simulink model "FullCardioLablModel"  (R2023b)
settings: Solver=FixedStepDiscrete  StartTime=0.0  StopTime=param_sim_time  FixedStep=1/fs  MaxStep=1/fs  RelTol=1e-3
undefined symbols (not defined in the file): analyses, fdesignblkfcn, fs, gcbh, param_tot_samples
libraries: dspstat3 x13, SCGAnalysis_SignalGenerationLib x2
(part 13 of 20)

== matlab function FullCardioLablModel/SCG Analysis/Enabled SCG Analysis Subsystem/All Signals Signal Metric Characterization/SCG 3DMinS2p2pProjection Signal Metric Characterization/Spectral Distribution Calculator/Spectral Distribution Calculator ==
  data: fs input size=[1]; r_pos input; scg_signal input; entire_cycle_nsd output size=[3 1]; entire_cycle_flag input size=[1]; s1_flag input size=[1]; s2_flag input size=[1]; f_band_lo input size=[1 2]; f_band_mid input size=[1 2]; f_band_hi input size=[1 2]; s1_nsd output size=[3 1]; s2_nsd output size=[3 1]
function [entire_cycle_nsd, s1_nsd, s2_nsd] = slk_normalized_spectral_distribution_calculator(fs, r_pos,scg_signal, entire_cycle_flag, s1_flag, s2_flag, f_band_lo, f_band_mid, f_band_hi)
% Simulink function to calculate the normalized spectral distribution of the power spectral densities of the entire cyle, the s1 complex, and the s2 complex, of an input SCG signal.

% INPUTS:
% fs = sampling frequency of scg_signal.
% r_pos = index positions of the R peaks of the ecg.
% scg_signal = signal to calculate its average cycle.
% entire_cycle_flag = flag to indicate the calculation of the entire cycle spectral distribution.
% s1_flag = flag to indicate the calculation of the S1 complex spectral distribution.
% s2_flag = flag to indicate the calculation of the S2 complex spectral distribution.

% OUTPUT:
% entire_cycle_nsd = normalized spectral distribution of the entire cycle (given as 3 elements corresponding to the spectral distribution in each of the 3 bins).
% s1_nsd = normalized spectral distribution of the s1 complex (given as 3 elements corresponding to the spectral distribution in each of the 3 bins).
% s2_nsd = normalized spectral distribution of the s2 complex (given as 3 elements corresponding to the spectral distribution in each of the 3 bins).

% This function consists of three parts:
% Part 1 - Calculation of the entire cycle normalized spectral distribution.
% Part 2 - Calculation of the S1 complex normalized spectral distribution.
% Part 3 - Calculation of the S2 complex normalized spectral distribution.

coder.extrinsic('legend');
coder.extrinsic('vline');

num_cycles = length(r_pos);

pad_size = 10*fs; % The length of the zero-padded vector used to obtain sufficient frequency resolution for the FFT.

PSDs = figure;
xlabel('Frequency (Hz)')
ylabel('Power Spectral Density (mg^2)')
xlim([0 f_band_hi(2)])
title('Power Spectral Densities')
hold on

freq_axis = fs*(0:pad_size/2)/pad_size; % Frequency axis for the FFT.

%% Part 1 - Calculation of the entire cycle normalized spectral distribution.


% if entire_cycle_flag
%     
%     current_cycle_padded = zeros(pad_size,1); % Pre-initializing for speed.
%     fft_entire_cycle_mag_2_sided = zeros(pad_size,1);
%     fft_entire_cycle_mag_1_sided = zeros(pad_size/2+1,num_cycles - 1);
%     
%     for i = 1:num_cycles - 1 % The last cycle isnt considered because it's not complete.
%         
%         current_cycle = scg_signal(r_pos(i):r_pos(i+1));
%         current_cycle_length = length(current_cycle); % In samples.
%         
%         % Ensuring the current cycle has an even number of samples - necessary for FFT calculation.
%         if mod(current_cycle_length,2) > 0
%             current_cycle_length = current_cycle_length - 1;
%             current_cycle(end) = [];
%         end
%                
%         current_cycle_padded = [current_cycle; zeros(pad_size - current_cycle_length,1)];
%         fft_entire_cycle = fft(current_cycle_padded); % (Complex) FFT values.
%         fft_entire_cycle_mag_2_sided = abs(fft_entire_cycle); % Two-sided Magnitude.
%         fft_entire_cycle_mag_1_sided(:,i) = fft_entire_cycle_mag_2_sided(1:length(current_cycle_padded)/2+1); % One-sided Magnitude.
%         fft_entire_cycle_mag_1_sided(2:end-1,i) = 2*fft_entire_cycle_mag_1_sided(2:end-1,i); % Multiplying by 2 to get total power (negative + positive frequencies).
%     end
%     
%     average_entire_cycle_fft = mean(fft_entire_cycle_mag_1_sided'); % The mean magnitude FFT spectrum.
%     
%     average_entire_cycle_psd = average_entire_cycle_fft.^2; % The power spectral density - the square of the magnitude spectrum.
%     
%     % Plotting.
%     figure(PSDs); hold on;
%     plot(freq_axis,average_entire_cycle_psd)
%     
%     % Integrating along the bands to get the bandpower.
%     entire_cycle_lo_power = trapz(ceil(f_band_lo(1)/freq_axis(2)):ceil(f_band_lo(2)/freq_axis(2)),average_entire_cycle_psd(ceil(f_band_lo(1)/freq_axis(2)):ceil(f_band_lo(2)/freq_axis(2))));
%     entire_cycle_mid_power = trapz(ceil(f_band_mid(1)/freq_axis(2)):ceil(f_band_mid(2)/freq_axis(2)),average_entire_cycle_psd(ceil(f_band_mid(1)/freq_axis(2)):ceil(f_band_mid(2)/freq_axis(2))));
%     entire_cycle_hi_power = trapz(ceil(f_band_hi(1)/freq_axis(2)):ceil(f_band_hi(2)/freq_axis(2)),average_entire_cycle_psd(ceil(f_band_hi(1)/freq_axis(2)):ceil(f_band_hi(2)/freq_axis(2))));
%     entire_cycle_total_power = trapz(ceil(f_band_lo(1)/freq_axis(2)):ceil(f_band_hi(2)/freq_axis(2)),average_entire_cycle_psd(ceil(f_band_lo(1)/freq_axis(2)):ceil(f_band_hi(2)/freq_axis(2))));
%     
%     % Dividing over total power to get the normalized spectral distribution (NSD).
%     normalized_entire_cycle_lo_power = entire_cycle_lo_power/entire_cycle_total_power;
%     normalized_entire_cycle_mid_power = entire_cycle_mid_power/entire_cycle_total_power;
%     normalized_entire_cycle_hi_power = entire_cycle_hi_power/entire_cycle_total_power;
%     
%     % Preparing outputs.
%     entire_cycle_nsd = [normalized_entire_cycle_lo_power;normalized_entire_cycle_mid_power;normalized_entire_cycle_hi_power];
%     
% else 
%     entire_cycle_nsd = [0; 0; 0];
% end


if entire_cycle_flag

    Interp_FFT_Cycle_Mag_1_Sided = zeros(num_cycles - 1, 10000); % Pre-initializing for speed.
    new_freq_axis_entire_cycle = linspace(0,fs/2,10000); % Interpolation frequency axis.

    for i = 1:num_cycles - 1 % The last cycle isnt considered because it's not complete.

        current_cycle = scg_signal(r_pos(i):r_pos(i+1));
        current_cycle_length = length(current_cycle); % In samples.

        % Ensuring the current cycle has an even number of samples - necessary for FFT calculation.
        if mod(current_cycle_length,2) > 0
            current_cycle_length = current_cycle_length - 1;
            current_cycle(end) = [];
        end

        FFT_Cycle = zeros(current_cycle_length,1); % Pre-initializing for speed.
        FFT_Cycle_Mag_2_Sided = zeros(current_cycle_length,1);
        FFT_Cycle_Mag_1_Sided = zeros(current_cycle_length/2+1,1);

        freq_axis_entire_cycle = fs*(0:current_cycle_length/2)/current_cycle_length; % Frequency axis for the FFT.

        % FFT of each individual cycle.
        FFT_Cycle = fft(current_cycle); % (Complex) FFT values.
        FFT_Cycle_Mag_2_Sided = abs(FFT_Cycle); % Two-sided Magnitude.
        FFT_Cycle_Mag_1_Sided = FFT_Cycle_Mag_2_Sided(1:current_cycle_length/2+1); % One-sided Magnitude.
        FFT_Cycle_Mag_1_Sided(2:end-1) = 2*FFT_Cycle_Mag_1_Sided(2:end-1); % Multiplying by 2 to get total power (negative + positive frequencies).

        % Interpolating to a new frequency axis. This is necessary because different cycles have different lenghts (and thus different FFT
        % lengths). To average the FFT across cycles, these must be interpolated to a particular fixed length.
        Interp_FFT_Cycle_Mag_1_Sided(i,:) = interp1(freq_axis_entire_cycle, FFT_Cycle_Mag_1_Sided, new_freq_axis_entire_cycle);

    end

    average_entire_cycle_FFT = mean(Interp_FFT_Cycle_Mag_1_Sided); % The mean magnitude FFT spectrum.

    average_entire_cycle_PSD = average_entire_cycle_FFT.^2; % The power spectral density - the square of the magnitude spectrum.

    % Plotting
    figure(PSDs);
    plot(new_freq_axis_entire_cycle,average_entire_cycle_PSD)

    % Integrating along the bands to get the bandpower.
    entire_cycle_lo_power = trapz(ceil(f_band_lo(1)/new_freq_axis_entire_cycle(2)):ceil(f_band_lo(2)/new_freq_axis_entire_cycle(2)),average_entire_cycle_PSD(ceil(f_band_lo(1)/new_freq_axis_entire_cycle(2)):ceil(f_band_lo(2)/new_freq_axis_entire_cycle(2))));
    entire_cycle_mid_power = trapz(ceil(f_band_mid(1)/new_freq_axis_entire_cycle(2)):ceil(f_band_mid(2)/new_freq_axis_entire_cycle(2)),average_entire_cycle_PSD(ceil(f_band_mid(1)/new_freq_axis_entire_cycle(2)):ceil(f_band_mid(2)/new_freq_axis_entire_cycle(2))));
    entire_cycle_hi_power = trapz(ceil(f_band_hi(1)/new_freq_axis_entire_cycle(2)):ceil(f_band_hi(2)/new_freq_axis_entire_cycle(2)),average_entire_cycle_PSD(ceil(f_band_hi(1)/new_freq_axis_entire_cycle(2)):ceil(f_band_hi(2)/new_freq_axis_entire_cycle(2))));
    entire_cycle_total_power = trapz(ceil(f_band_lo(1)/new_freq_axis_entire_cycle(2)):ceil(f_band_hi(2)/new_freq_axis_entire_cycle(2)),average_entire_cycle_PSD(ceil(f_band_lo(1)/new_freq_axis_entire_cycle(2)):ceil(f_band_hi(2)/new_freq_axis_entire_cycle(2))));

    % Dividing over total power to get the normalized spectral distribution (NSD).
    normalized_entire_cyce_lo_power = entire_cycle_lo_power/entire_cycle_total_power;
    normalized_entire_cyce_mid_power = entire_cycle_mid_power/entire_cycle_total_power;
    normalized_entire_cyce_hi_power = entire_cycle_hi_power/entire_cycle_total_power;

    % Preparing outputs.
    entire_cycle_nsd = [normalized_entire_cyce_lo_power;normalized_entire_cyce_mid_power;normalized_entire_cyce_hi_power];

    
else 
    entire_cycle_nsd = [0; 0; 0];

end

%% Part 2 - Calculation of the S1 complex normalized spectral distribution.

if s1_flag
    
    s1 = zeros(0.2*fs,1); % Pre-initializing for speed.
    s1_padded = zeros(pad_size,1);
    fft_s1_mag_2_sided = zeros(pad_size,1);
    fft_s1_mag_1_sided = zeros((pad_size)/2+1,num_cycles - 1);
    
    for i = 1:num_cycles - 1 % The last cycle isnt considered because there is a chance its S1 complex will be cut.
        s1 = scg_signal(r_pos(i):r_pos(i) + 0.2*fs - 1); % The S1 complex is considered as the 200ms following the ECG R peak.
        s1_padded = [s1; zeros(pad_size - 0.2*fs,1)];
        fft_s1 = fft(s1_padded); % (Complex) FFT values.
        fft_s1_mag_2_sided = abs(fft_s1); % Two-sided Magnitude.
        fft_s1_mag_1_sided(:,i) = fft_s1_mag_2_sided(1:length(s1_padded)/2+1); % One-sided Magnitude.
        fft_s1_mag_1_sided(2:end-1,i) = 2*fft_s1_mag_1_sided(2:end-1,i); % Multiplying by 2 to get total power (negative + positive frequencies).
    end
    
    average_s1_fft = mean(fft_s1_mag_1_sided'); % The mean magnitude FFT spectrum.
    
    average_s1_psd = average_s1_fft.^2; % The power spectral density - the square of the magnitude spectrum.
    
    % Plotting.
    figure(PSDs); hold on
    plot(freq_axis,average_s1_psd)
    
    % Integrating along the bands to get the bandpower.
    s1_lo_power = trapz(ceil(f_band_lo(1)/freq_axis(2)):ceil(f_band_lo(2)/freq_axis(2)),average_s1_psd(ceil(f_band_lo(1)/freq_axis(2)):ceil(f_band_lo(2)/freq_axis(2))));
    s1_mid_power = trapz(ceil(f_band_mid(1)/freq_axis(2)):ceil(f_band_mid(2)/freq_axis(2)),average_s1_psd(ceil(f_band_mid(1)/freq_axis(2)):ceil(f_band_mid(2)/freq_axis(2))));
    s1_hi_power = trapz(ceil(f_band_hi(1)/freq_axis(2)):ceil(f_band_hi(2)/freq_axis(2)),average_s1_psd(ceil(f_band_hi(1)/freq_axis(2)):ceil(f_band_hi(2)/freq_axis(2))));
    s1_total_power = trapz(ceil(f_band_lo(1)/freq_axis(2)):ceil(f_band_hi(2)/freq_axis(2)),average_s1_psd(ceil(f_band_lo(1)/freq_axis(2)):ceil(f_band_hi(2)/freq_axis(2))));
    
    % Dividing over total power to get the normalized spectral distribution (NSD).
    normalized_s1_lo_power = s1_lo_power/s1_total_power;
    normalized_s1_mid_power = s1_mid_power/s1_total_power;
    normalized_s1_hi_power = s1_hi_power/s1_total_power;
    
    % Preparing outputs.
    s1_nsd = [normalized_s1_lo_power;normalized_s1_mid_power;normalized_s1_hi_power];
    
else
    s1_nsd = [0; 0; 0;];
end

%% Part 3 - Calculation of the S2 complex normalized spectral distribution.

if s2_flag
    
    s2_search_window_lims = [0.25*fs 0.5*fs]; % The window initially used to search for the S2 peak within that cycle.
    s2_identify_window = 0.15*fs; % The window length centered about the S2 peak (in samples) used to identify the S2 complex.
    
    s2 = zeros(s2_identify_window,1); % Pre-initializing for speed.
    s2_padded = zeros(pad_size,1);
    fft_s2_mag_2_sided = zeros(pad_size,1);
    fft_s2_mag_1_sided = zeros((pad_size)/2+1,num_cycles - 1);
    
    for i = 1:num_cycles - 1 % The last cycle isnt considered because there is a chance its S1 complex will be cut.
        
        cycle = scg_signal(r_pos(i):r_pos(i+1)); % The current heart cycle.
        
        s2_search_window = cycle(s2_search_window_lims(1):s2_search_window_lims(2)); % Defining the window where to search for the S2 peak.
        s2peak = s2_search_window_lims(1) + find(abs(s2_search_window)==max(abs(s2_search_window))); % Identifying the S2 peak within 'cycle'.
        
        s2 = cycle(s2peak(1) - s2_identify_window/2 : s2peak(1) + s2_identify_window/2); % The S2 complex.
        s2_padded = [s2; zeros(pad_size - s2_identify_window - 1,1)]; % Padding the S2 complex with zeros.
        fft_s2 = fft(s2_padded); % (Complex) FFT values.
        fft_s2_mag_2_sided = abs(fft_s2); % Two-sided Magnitude.
        fft_s2_mag_1_sided(:,i) = fft_s2_mag_2_sided(1:length(s2_padded)/2+1); % One-sided Magnitude.
        fft_s2_mag_1_sided(2:end-1,i) = 2*fft_s2_mag_1_sided(2:end-1,i); % Multiplying by 2 to get total power (negative + positive frequencies).
    end
    
    average_s2_FFT = mean(fft_s2_mag_1_sided'); % The mean magnitude FFT spectrum.
    
    average_s2_PSD = average_s2_FFT.^2; % The power spectral density - the square of the magnitude spectrum.
    
    % Plotting.
    figure(PSDs); hold on;
    title('SCG 3D Systolic Min S2p2p Axis')
    plot(freq_axis,average_s2_PSD)
    
    % Integrating along the bands to get the bandpower.
    s2_lo_power = trapz(ceil(f_band_lo(1)/freq_axis(2)):ceil(f_band_lo(2)/freq_axis(2)),average_s2_PSD(ceil(f_band_lo(1)/freq_axis(2)):ceil(f_band_lo(2)/freq_axis(2))));
    s2_mid_power = trapz(ceil(f_band_mid(1)/freq_axis(2)):ceil(f_band_mid(2)/freq_axis(2)),average_s2_PSD(ceil(f_band_mid(1)/freq_axis(2)):ceil(f_band_mid(2)/freq_axis(2))));
    s2_hi_power = trapz(ceil(f_band_hi(1)/freq_axis(2)):ceil(f_band_hi(2)/freq_axis(2)),average_s2_PSD(ceil(f_band_hi(1)/freq_axis(2)):ceil(f_band_hi(2)/freq_axis(2))));
    s2_total_power = trapz(ceil(f_band_lo(1)/freq_axis(2)):ceil(f_band_hi(2)/freq_axis(2)),average_s2_PSD(ceil(f_band_lo(1)/freq_axis(2)):ceil(f_band_hi(2)/freq_axis(2))));
    
    % Dividing over total power to get the normalized spectral distribution (NSD).
    normalized_s2_lo_power = s2_lo_power/s2_total_power;
    normalized_s2_mid_power = s2_mid_power/s2_total_power;
    normalized_s2_hi_power = s2_hi_power/s2_total_power;
    
    % Preparing outputs.
    s2_nsd = [normalized_s2_lo_power;normalized_s2_mid_power;normalized_s2_hi_power];
    
else 
    s2_nsd = [0;0;0];    
end

% Plotting the frequency band delimiters
vline(f_band_lo(1),'r')
vline(f_band_mid(1),'r')
vline(f_band_hi(1),'r')
vline(f_band_hi(2),'r')

% Plotting the legend.
if entire_cycle_flag
    legend('Entire Cycle')
end

if s1_flag
    legend('S1')
end

if s2_flag
    legend('S2')
end

if entire_cycle_flag && s1_flag
    legend('Entire Cycle','S1')
end

if entire_cycle_flag && s2_flag
    legend('Entire Cycle','S2')
end

if s1_flag && s2_flag
    legend('S1','S2')
end

if entire_cycle_flag && s1_flag && s2_flag
    legend('Entire Cycle','S1','S2')
end

end

== matlab function FullCardioLablModel/SCG Analysis/Enabled SCG Analysis Subsystem/Systolic Interval Identification/Systolic Fiducial Point Marker/3D Systolic Fiducial Point Identifier ==
  data: fs input size=[1]; MC output size=[4*ceil(param_sim_time) 1]; MC_prelim input; IM_prelim input; IM output size=[4*ceil(param_sim_time) 1]; AO output size=[4*ceil(param_sim_time) 1]; AO_prelim input; scg_s1_3DMod input
function [MC, IM, AO] = slk_3D_systolic_fiducial_point_identifier(fs, MC_prelim, IM_prelim, AO_prelim, scg_s1_3DMod)
% Function to identify the (final) systolic hemodynamic fiducial points of the seismocardiogram (SCG) based on the preliminary systolic markers and using an S1 3D modulus signal.

% INPUTS:
% fs - the sampling frequency (in Hz).
% MC_prelim - preliminary sample indexes of mitral closure.
% IM_prelim - preliminary sample indexes isovolumic moment.
% AO_prelim_ - preliminary sample indexes of aortic opening.
% scg_s1_3DMod - the systolic (i.e, constructed from the S1 bandwidth-optimized x,y,z SCG components) 3DModulus signal.

% OUTPUTS:
% MC - final sample indexes of mitral closure.
% IM - final sample indexes isovolumic moment.
% AO - final sample indexes of aortic opening.

coder.extrinsic('legend');

% Plotting before refining.
Labelled3DSCG = figure;
plot(scg_s1_3DMod); hold on;
plot(IM_prelim, scg_s1_3DMod(IM_prelim),'xr')
plot(MC_prelim, scg_s1_3DMod(MC_prelim),'xb')
plot(AO_prelim, scg_s1_3DMod(AO_prelim),'xk')
box off

title('Systolic Fiducial Markers')
xlabel('Sample no.')
ylabel('Acceleration (mg)')

IM = zeros(length(IM_prelim), 1);   % Pre-initalization for speed.
MC = zeros(length(MC_prelim), 1);
AO = zeros(length(AO_prelim), 1);

MC_search_window_size = fs*0.02; % The window centered about MC_prelim where we will search for MC in the 3D Mod signal.
IM_search_window_size = fs*0.02; % The window centered about MC_prelim where we will search for MC in the 3D Mod signal.
AO_search_window_size = fs*0.04; % The window centered about MC_prelim where we will search for MC in the 3D Mod signal.


% Refining MC
for i = 1:length(MC_prelim)
    
    MC_search_window = scg_s1_3DMod(MC_prelim(i) - floor(MC_search_window_size/2):MC_prelim(i) + ceil(MC_search_window_size/2));
    [MC_candies_amps, MC_candies_locs, MC_candies_widths, MC_candies_proms]  = findpeaks(MC_search_window); % Identifying the amplitude, location, width, and prominence of the detected peaks.
    
    if MC_candies_amps % If peaks were detected...
        %MC_candy = MC_candies_locs(find(MC_candies_amps == max(MC_candies_amps))); % Consider MC as the peak with the maximum amplitude.
        %MC_candy = MC_candies_locs(1); % Consider MC as the first peak
        %MC_candy = MC_candies_locs(find(MC_candies_widths == max(MC_candies_widths))); % Consider MC as the peak with the greatest width.
        MC_candy = MC_candies_locs(find(MC_candies_proms == max(MC_candies_proms))); % Consider MC as the peak with the maximum prominence.
        MC(i) = -1 + MC_prelim(i) - floor(MC_search_window_size/2) + MC_candy;
    else
        MC(i) = nan;
    end
    
    MC_candy = []; % Clearing.
    MC_candies_amps = [];
    MC_candies_locs = [];
    MC_candies_widths = [];
    MC_candies_proms = [];
    
end

% Refining IM
for i = 1:length(IM_prelim)
    
    IM_search_window = scg_s1_3DMod(IM_prelim(i) - floor(IM_search_window_size/2):IM_prelim(i) + ceil(IM_search_window_size/2));
    [IM_candies_amps, IM_candies_locs, IM_candies_widths, IM_candies_proms]  = findpeaks(IM_search_window); % Identifying the amplitude, location, width, and prominence of the detected peaks.
    
    if IM_candies_amps % If peaks were detected...
        %IM_candy = IM_candies_locs(find(IM_candies_amps == max(IM_candies_amps))); % Consider IM as the peak with the maximum amplitude.
        %IM_candy = IM_candies_locs(1); % Consider IM as the first peak
        %IM_candy = IM_candies_locs(find(IM_candies_widths == max(IM_candies_widths))); % Consider IM as the peak with the greatest width.
        IM_candy = IM_candies_locs(find(IM_candies_proms == max(IM_candies_proms))); % Consider IM as the peak with the maximum prominence.
        IM(i) = -1 + IM_prelim(i) - floor(IM_search_window_size/2) + IM_candy;
    else
        IM(i) = nan;
    end
    
    IM_candy = []; % Clearing.
    IM_candies_amps = [];
    IM_candies_locs = [];
    IM_candies_widths = [];
    IM_candies_proms = [];
    
end

% Refining AO
for i = 1:length(AO_prelim)
    
    AO_lower_search_lim = max([IM(i), AO_prelim(i) - floor(AO_search_window_size/2)]); % Making sure the serach window does not include the IM peak.
    
    AO_search_window = scg_s1_3DMod(AO_lower_search_lim : AO_prelim(i) + ceil(AO_search_window_size/2));
    [AO_candies_amps, AO_candies_locs, AO_candies_widths, AO_candies_proms]  = findpeaks(AO_search_window); % Identifying the amplitude, location, width, and prominence of the detected peaks.
    
    if AO_candies_amps % If peaks were detected...
        %AO(i) = AO_candies_locs(find(AO_candies_amps == max(AO_candies_amps))); % Consider AO as the peak with the maximum amplitude.
        AO_candy = AO_candies_locs(1); % Consider AO as the first peak
        %AO_candy = AO_candies_locs(find(AO_candies_widths == max(AO_candies_widths))); % Consider AO as the peak with the greatest width.
        %AO_candy = AO_candies_locs(find(AO_candies_proms == max(AO_candies_proms))); % Consider AO as the peak with the maximum prominence.
        AO(i) = -1 + AO_lower_search_lim + AO_candy;
    else
        AO(i) = nan;
    end
    
    AO_candy = []; % Clearing.
    AO_candies_amps = [];
    AO_candies_locs = [];
    AO_candies_widths = [];
    AO_candies_proms = [];
    AO_lower_search_lim = [];
    
end

figure(Labelled3DSCG);
hold on;
plot(IM(~isnan(IM)), scg_s1_3DMod(IM(~isnan(IM))),'or') % Do not plot the 'nans'.
plot(MC(~isnan(MC)), scg_s1_3DMod(MC(~isnan(MC))),'ob')
plot(AO(~isnan(AO)), scg_s1_3DMod(AO(~isnan(AO))),'ok')

legend('3D Modulus','IM_p_r_e_l_i_m','MC_p_r_e_l_i_m','AO_p_r_e_l_i_m','IM','MC','AO')

end

== matlab function FullCardioLablModel/SCG Analysis/Enabled SCG Analysis Subsystem/Systolic Interval Identification/Diastolic Fiducial Point Marker/3D Diastolic Fiducial Point Identifier ==
  data: fs input size=[1]; AC output size=[4*ceil(param_sim_time) 1]; AC_prelim input; MO_prelim input; MO output size=[4*ceil(param_sim_time) 1]; scg_s2_3DMod input
function [AC, MO] = slk_3D_diastolic_fiducial_point_identifier(fs, AC_prelim, MO_prelim, scg_s2_3DMod)
% Function to identify the (final) diastolic hemodynamic fiducial points of the seismocardiogram (SCG) based on the preliminary diastolic markers and using an S2 3D modulus signal.

% INPUTS:
% fs - the sampling frequency (in Hz).
% AC_prelim - preliminary sample indexes of aortic closure.
% MO_prelim - preliminary sample indexes mitral opening.
% scg_s2_3DMod - the diastolic (i.e, constructed from the S2 bandwidth-optimized x,y,z SCG components) 3DModulus signal.

% OUTPUTS:
% AC - final sample indexes of aortic opening.
% MO - final sample indexes of mitral opening.

coder.extrinsic('legend');

% Plotting before refining.
Labelled3DSCG = figure;
plot(scg_s2_3DMod); hold on;
plot(AC_prelim(~isnan(AC_prelim)), scg_s2_3DMod(AC_prelim(~isnan(AC_prelim))),'xb') % Do not plot the 'nans'.
plot(MO_prelim(~isnan(MO_prelim)), scg_s2_3DMod(MO_prelim(~isnan(MO_prelim))),'xr')
box off

title('Diastolic Fiducial Markers')
xlabel('Sample no.')
ylabel('Acceleration (mg)')

AC = zeros(length(MO_prelim), 1);   % Pre-initalization for speed.
MO = zeros(length(AC_prelim), 1);


AC_search_window_size = fs*0.02; % The window centered about AC_prelim where we will search for AC in the 3D Mod signal.
MO_search_window_size = fs*0.02; % The window centered about MO_prelim where we will search for MO in the 3D Mod signal.


% Refining AC
for i = 1:length(AC_prelim)
    
    if isnan(AC_prelim(i))
        
        AC(i) = nan;

    else
        
        AC_search_window = scg_s2_3DMod(AC_prelim(i) - floor(AC_search_window_size/2):AC_prelim(i) + ceil(AC_search_window_size/2));
        [AC_candies_amps, AC_candies_locs, AC_candies_widths, AC_candies_proms]  = findpeaks(AC_search_window); % Identifying the amplitude, location, width, and prominence of the detected peaks.
        
        if AC_candies_amps % If peaks were detected...
            %AC_candy = MC_candies_locs(find(MC_candies_amps == max(MC_candies_amps)));      % Consider AC as the peak with the maximum amplitude.
            %AC_candy = MC_candies_locs(1);                                                  % Consider AC as the first peak.
            %AC_candy = MC_candies_locs(find(MC_candies_widths == max(MC_candies_widths)));  % Consider AC as the peak with the greatest width.
            AC_candy = AC_candies_locs(find(AC_candies_proms == max(AC_candies_proms)));     % Consider AC as the peak with the maximum prominence.
            AC(i) = -1 + AC_prelim(i) - floor(AC_search_window_size/2) + AC_candy;
        else
            AC(i) = nan;
        end
        
        AC_candy = []; % Clearing.
        AC_candies_amps = [];
        AC_candies_locs = [];
        AC_candies_widths = [];
        AC_candies_proms = [];
        
    end
end

% Refining MO
for i = 1:length(MO_prelim)
    
    if isnan(MO_prelim(i))
        
        MO(i) = nan;
        
    else
        
        MO_search_window = scg_s2_3DMod(MO_prelim(i) - floor(MO_search_window_size/2):MO_prelim(i) + ceil(MO_search_window_size/2));
        [MO_candies_amps, MO_candies_locs, MO_candies_widths, MO_candies_proms]  = findpeaks(MO_search_window); % Identifying the amplitude, location, width, and prominence of the detected peaks.
        
        if MO_candies_amps % If peaks were detected...
            %MO_candy = IM_candies_locs(find(MO_candies_amps == max(MO_candies_amps)));       % Consider MO as the peak with the maximum amplitude.
            %MO_candy = IM_candies_locs(1);                                                   % Consider MO as the first peak
            %MO_candy = IM_candies_locs(find(IM_candies_widths == max(IM_candies_widths)));   % Consider MO as the peak with the greatest width.
            MO_candy = MO_candies_locs(find(MO_candies_proms == max(MO_candies_proms)));     % Consider MO as the peak with the maximum prominence.
            MO(i) = -1 + MO_prelim(i) - floor(MO_search_window_size/2) + MO_candy;
        else
            AC(i) = nan;
        end
        
        MO_candy = []; % Clearing.
        MO_candies_amps = [];
        MO_candies_locs = [];
        MO_candies_widths = [];
        MO_candies_proms = [];
        
    end
    
end

figure(Labelled3DSCG);
hold on;
plot(AC(~isnan(AC)), scg_s2_3DMod(AC(~isnan(AC))),'ob') % Do not plot the 'nans'.
plot(MO(~isnan(MO)), scg_s2_3DMod(MO(~isnan(MO))),'or')

legend('3D Modulus','AC_p_r_e_l_i_m','MO_p_r_e_l_i_m','AC','MO')

end

== matlab function FullCardioLablModel/ECG Analysis/Enabled ECG Analysis Subsystem/Assign To Workspace: Num Cycles/Enabled To Workspace ECG Num Cycles/Slk Wrapped Assigned To Workspace ==
  data: assigned_var input size=[1]
function slk_wrapped_assign_to_workspace(assigned_var)
% Wrapped simulink function to assign an input 'assigned_var' to the base workspace.

coder.extrinsic('assign_num_cycles_to_workspace');

if assigned_var % Only go into the function if a valid variable is passed to it.
    assign_num_cycles_to_workspace(assigned_var)
end

end

== matlab function FullCardioLablModel/SCG Analysis/Enabled SCG Analysis Subsystem/Systolic Interval Identification/Diastolic Fiducial Point Marker/Preliminary Diastolic Fiducial Point Identifier ==
  data: fs input size=[1]; AC_prelim output size=[4*ceil(param_sim_time) 1]; ecg_r_pos input; ecg_t_pos input; MO_prelim output size=[4*ceil(param_sim_time) 1]; scg_s2_ref_signal input
function [AC_prelim, MO_prelim] = slk_preliminary_diastolic_fiducial_point_identifier(fs, ecg_r_pos, ecg_t_pos, scg_s2_ref_signal)
% Function to identify the (preliminary) diastolic hemodynamic fiducial points of the seismocardiogram (SCG) using an s2 reference signal.

% To identify the S2 location, the T wave peaks are used. If these are not available, the R wave peaks are used instead.
% A first S2 anchor point is identified using the TKEO (the S2 complex is typically high frequency). Based on this anchor point, a second S2
% anchor point is identified as the trough of the SCG S2 reference signal closest to the first anchor. The preliminary S2 fiducial
% points (AC_prelim and MO_prelim), are then identified based on these S2 anchors. AC_prelim is the first peak immediately before the second S2
% anchor point. MO_prelim is the most prominent trough after tge second S2 anchor point.

% INPUTS:
% fs - the sampling frequency (in Hz).
% ecg_r_pos - the ECG R peaks.
% ecg_t_pos - the ECG T peaks.
% scg_s2_ref_signal - the SCG diastolic reference signal used to perform a preliminary identificaiton of the SCG diastolic fiducial points (ie. MC, IM, and AO).

% OUTPUTS:
% AC_prelim - preliminary sample indexes of aortic closure.
% MO_prelim - preliminary sample indexes mitral opening.

% NOTE - This code assumes coherent segmentation between the input R and T peaks (i.e. the nth T wave peak corresponds to the same cycle of the nth R wave peak such that r(i) < t(i) < r(i+1)).

coder.extrinsic('legend')

num_cycles = size(ecg_r_pos,1);

rr = diff(ecg_r_pos); % RR intervals (in samples).

% Defining search window limits.
if ecg_t_pos
    s2_1st_search_window_relative_lims = [-0.075 0.9]; % The lower and upper limits of the first S2 search window opened relative to the T peak (lower) and R peak (upper) and given as the portion of that cycle's RR interval. Hence, we are accounting for shorter cycles. If the first value is negative we look for the S2 starting BEFORE the T wave peak.
else
    s2_1st_search_window_relative_lims = [0.2 0.9]; % The lower and upper limits of the first S2 search window relative to the R peak and given as the portion of that cycle's RR interval. Hence, we are accounting for shorter cycles.
end

s2_2nd_search_window_lims = [-0.025*fs 0.0125*fs]; % The lower and upper limits of the second S2 search window opened with respect to the first S2 anchor point (i.e. the max S2 TKEO peak). This window is not RR-sensitive (it is given in absolute terms).
AC_prelim_search_window_lims = [-0.015*fs 0]; % The lower and upper limits of the AC_prelim search window opened with respect to the second S2 anchor point (i.e. the maximum trough preceding the first S1 anchor point). This window is not RR-sensitive (it is given in absolute terms).
MO_prelim_search_window_lims = [0 0.1*fs];

AC_prelim = zeros(num_cycles - 1 , 1);   % Pre-initalization of the outputs for speed.
MO_prelim = zeros(num_cycles - 1 , 1);

for i = 1:num_cycles - 1% The last cycle isn't considered because there's a good chance its SCG fiducial markers are cut off.
    
    cycle = scg_s2_ref_signal(ecg_r_pos(i):ecg_r_pos(i+1));
    tkeo_cycle = tkeo(cycle);
    
    if ecg_t_pos
        
        % FIRST ANCHOR - The peak of the TKEO in a S2 complex search window.
        s2_1st_search_window = tkeo_cycle( -1*ecg_r_pos(i) + ecg_t_pos(i) + floor(rr(i)*s2_1st_search_window_relative_lims(1)) : ceil(rr(i)*s2_1st_search_window_relative_lims(2))); % The first window to search for the first anchor with the TKEO signal.
        [s2_1st_anchor_candies_amps, s2_1st_anchor_candies_locs, s2_1st_anchor_candies_widths, s2_1st_anchor_candies_proms] = findpeaks(s2_1st_search_window); % The candidate (TKEO) peak amplitudes, locations, widths and prominences of the first S2 anchor.
        
    else
        
        % FIRST ANCHOR - The peak of the TKEO in a S2 complex search window.
        s2_1st_search_window = tkeo_cycle( -1*ecg_r_pos(i) + ecg_t_pos(i) + floor(rr(i)*s2_1st_search_window_relative_lims(1)) : ceil(rr(i)*s2_1st_search_window_relative_lims(2))); % The first window to search for the first anchor with the TKEO signal.
        [s2_1st_anchor_candies_amps, s2_1st_anchor_candies_locs, s2_1st_anchor_candies_widths, s2_1st_anchor_candies_proms] = findpeaks(s2_1st_search_window); % The candidate (TKEO) peak amplitudes, locations, widths and prominences of the first S2 anchor.
        
    end
    
    %s2_1st_anchor = s2_1st_anchor_candies_locs(find(s2_1st_anchor_candies_amps == max(s2_1st_anchor_candies_amps)));     % Consider the fisrt S2 anchor as the (TKEO) peak with the maximum amplitude.
    %s2_1st_anchor = s2_1st_anchor_candies_locs(1);                                                                       % Consider the first S2 anchor as the first (TKEO) peak.
    %s2_1st_anchor = s2_1st_anchor_candies_locs(find(s2_1st_anchor_candies_widths == max(s2_1st_anchor_candies_widths))); % Consider the first S2 anchor as the (TKEO)  peak with the greatest width.
    s2_1st_anchor = s2_1st_anchor_candies_locs(find(s2_1st_anchor_candies_proms == max(s2_1st_anchor_candies_proms)));    % Consider the first S2 anchor as the (TKEO) peak with the maximum prominence.
    
    s2_1st_anchor = -1 + s2_1st_anchor + floor(-1*ecg_r_pos(i) + ecg_t_pos(i) + rr(i)*s2_1st_search_window_relative_lims(1)); % Relocating S2 first anchor relative to 'cycle' start. The -1 adjusts for one-based indexing.
    
    % SECOND ANCHOR - The lowest trough close to the first anchor (mostly preceding it).
    s2_2nd_search_window = cycle(floor(s2_1st_anchor(1) + s2_2nd_search_window_lims(1)) : ceil(s2_1st_anchor(1) + s2_2nd_search_window_lims(2))); % The second window to search for the second anchor (the trough) in the original signal.
    [s2_2nd_anchor_candies_amps, s2_2nd_anchor_candies_locs, s2_2nd_anchor_candies_widths, s2_2nd_anchor_candies_proms] = findpeaks(-1*s2_2nd_search_window); % The candidate trough amplitudes, locations, widths and prominences of the second S2 anchor. The -1 flips the signal so the valleys are considered as peaks.
    
    s2_2nd_anchor = s2_2nd_anchor_candies_locs(find(s2_2nd_anchor_candies_amps == max(s2_2nd_anchor_candies_amps)));      % Consider the second S2 anchor as the valley with the lowest amplitude.
    %s2_2nd_anchor = s2_2nd_anchor_candies_locs(1);                                                                       % Consider the second S2 anchor as the first valley.
    %s2_2nd_anchor = s2_2nd_anchor_candies_locs(find(s2_2nd_anchor_candies_widths == max(s2_2nd_anchor_candies_widths))); % Consider the second S2 anchor as the valley with the greatest width.
    %s2_2nd_anchor = s2_2nd_anchor_candies_locs(find(s2_2nd_anchor_candies_proms == max(s2_2nd_anchor_candies_proms)));   % Consider the second S2 anchor as the valley with the maximum prominence.
    
    s2_2nd_anchor = -1 + s2_2nd_anchor + floor(s2_1st_anchor + s2_2nd_search_window_lims(1)); % Relocating S2 second anchor relative to 'cycle' start.
    
    % AC_prelim - The first peak immediately preceding the second anchor.
    AC_prelim_search_window = cycle(s2_2nd_anchor(1) + AC_prelim_search_window_lims(1) : s2_2nd_anchor(1) + + AC_prelim_search_window_lims(2));
    [AC_prelim_candies_amps, AC_prelim_candies_locs, AC_prelim_candies_widths, AC_prelim_candies_proms] = findpeaks(AC_prelim_search_window); % The candidate peak amplitudes, locations, widths and prominences of AC_prelim.
    
    if AC_prelim_candies_amps % If an AC_prelim was detected.
        %AC_prelim_local = AC_prelim_candies_locs(find(AC_prelim_candies_amps == max(AC_prelim_candies_amps)));     % Consider AC_prelim as the peak with the greatest amplitude.
        AC_prelim_local = AC_prelim_candies_locs(end);                                                              % Consider AC_prelim as the last peak (i.e. the one closest to the 2nd anchor).
        %AC_prelim_local = AC_prelim_candies_locs(find(AC_prelim_candies_widths == max(AC_prelim_candies_widths))); % Consider AC_prelim as the peak with the greatest width.
        %AC_prelim_local = AC_prelim_candies_locs(find(AC_prelim_candies_proms == max(AC_prelim_candies_proms)));   % Consider AC_prelim as the peak with the maximum prominence.
        
        AC_prelim(i) = -2 + ecg_r_pos(i) + floor(s2_2nd_anchor + AC_prelim_search_window_lims(1)) + AC_prelim_local; % Relocating AC_prelim with respect to the start of the recording. The -2 adjusts for 1-based indexing on two windowing operations.
    else
        AC_prelim(i) = nan;
    end
    
    %MO_prelim - The most significant trough after the second anchor.
    MO_prelim_search_window = cycle(s2_2nd_anchor(1) + MO_prelim_search_window_lims(1) : s2_2nd_anchor(1) + MO_prelim_search_window_lims(2));
    [MO_prelim_candies_amps, MO_prelim_candies_locs, MO_prelim_candies_widths, MO_prelim_candies_proms] = findpeaks(-1*MO_prelim_search_window); % The candidate trough amplitudes, locations, widths and prominences of AC_prelim. The -1 flips the signal so that the troughs are considered as peaks.
    
    if MO_prelim_candies_amps % If an MO_prelim was detected.
        %MO_prelim_local = MO_prelim_candies_locs(find(MO_prelim_candies_amps == max(MO_prelim_candies_amps)));     % Consider MO_prelim as the trough with the greatest amplitude.
        %MO_prelim_local = MO_prelim_candies_locs(1);                                                               % Consider MO_prelim as the first trough (i.e. the one closest to the 2nd anchor).
        %MO_prelim_local = MO_prelim_candies_locs(find(MO_prelim_candies_widths == max(MO_prelim_candies_widths))); % Consider MO_prelim as the trough with the greatest width.
        MO_prelim_local = MO_prelim_candies_locs(find(MO_prelim_candies_proms == max(MO_prelim_candies_proms)));    % Consider MO_prelim as the trough with the maximum prominence.
        
        MO_prelim(i) = -2 + ecg_r_pos(i) + floor(s2_2nd_anchor + MO_prelim_search_window_lims(1)) + MO_prelim_local; % Relocating MO_prelim with respect to the start of the recording. The -2 adjusts for 1-based indexing on two windowing operations.
    else
        MO_prelim(i) = nan;
    end 
    
    cycle = []; % Clearing.
    tkeo_cycle = [];
    s2_1st_search_window = []; 
    s2_1st_anchor = [];
    s2_2nd_search_window = [];
    s2_2nd_anchor = [];
    AC_prelim_search_window = [];
    AC_prelim_local = []; 
    MO_prelim_local = [];
    
end

% Plotting
t = 0:1/fs:(length(scg_s2_ref_signal)-1)/fs;

figure;
plot(t,scg_s2_ref_signal); hold on;
plot((AC_prelim(~isnan(AC_prelim))-1)/fs, scg_s2_ref_signal(AC_prelim(~isnan(AC_prelim))),'or') % Do not plot the 'nans'.
plot((MO_prelim(~isnan(MO_prelim))-1)/fs, scg_s2_ref_signal(MO_prelim(~isnan(MO_prelim))),'ob')

legend('SCG S2 Reference Signal','AC_p_r_e_l_i_m','MO_p_r_e_l_i_m')

box off

title('Preliminary Diastolic Fiducial Markers')
xlabel('Time (sec)')
ylabel('Acceleration (mg)')

end

== matlab function FullCardioLablModel/SCG Analysis/Enabled SCG Analysis Subsystem/Systolic Interval Identification/Average Calculator/slk_average_calculator ==
  data: average_type input size=[1]; series input; average output size=[1]
function average = slk_average_calculator(average_type, series)
% Simple function to return the user-defined average of an input series.

average = 0; % Pre-initialization

if average_type == 1
    average = mean(series(~isnan(series)));
elseif average_type == 2
    average = median(series(~isnan(series)));
elseif average_type == 3
    average = mode(series(~isnan(series)));
end

end

== matlab function FullCardioLablModel/SCG Analysis/Enabled SCG Analysis Subsystem/Systolic Interval Identification/MATLAB Function ==
  data: PEP output size=[4*ceil(param_sim_time) 1]; fs input size=[1]; IVC output size=[4*ceil(param_sim_time) 1]; ecg_q input; ecg_r input; ecg_t input; MC input; AO input; AC input; MO input; ET output size=[4*ceil(param_sim_time) 1]; IVR output size=[4*ceil(param_sim_time) 1]; DC output size=[4*ceil(param_sim_time) 1]
function [PEP, IVC, ET, IVR, DC]  = slk_cardiac_interval_identifier(fs, ecg_q, ecg_r, ecg_t, MC, AO, AC, MO)
% Function to calculate various cardiac intervals based on the previously-identified systolic and diastolic fiducial markers.

% INPUTS
% fs = sampling frequency.
% ecg_q = Q peak indices of the ECG.
% ecg_r = R peak indices of the ECG.
% MC = Mitral Closure indices of the SCG.
% IM = Isovolumic Moment indices of the SCG.
% AO = Aortic Opening indices of the SCG.
% MC = Mitral Closure indices of the SCG.

% OUTPUTS
% PEP = Pre-Ejection Period indices.
% IVC = Isovolumic Contraction indices.
% EJ = Ejection Time indices.
% IVR = Isovolumic Relaxation indices.

num_cycles = length(ecg_r) - 1; % Remember, the last cycle was not considered for systolic and diastolic fiducial point identification. 

IVC = zeros(num_cycles, 1); % Pre-initialization for speed.
PEP = zeros(num_cycles, 1);
ET = zeros(num_cycles, 1);
IVR = zeros(num_cycles, 1);
DC = zeros(num_cycles, 1);

for i = 2:num_cycles % We also don't consider the first cycle because there are often misdetections in the Q complex.
    
    %PEP (AO - Q or AO - R).
    if ecg_q(i) && ~isnan(AO(i))
        PEP(i) = (AO(i) - ecg_q(i))/fs;
    elseif ecg_r(i) && ~isnan(AO(i))
        PEP(i) = (AO(i) - ecg_q(i))/fs;
    else
        PEP(i) = nan;
    end
        
    %IVC (AO - MC).
    if ~isnan(MC(i)) && ~isnan(AO(i))
        IVC(i) = (AO(i) - MC(i))/fs;
    else
        IVC(i) = nan;
    end
    
    %ET (AC - AO).
    if ~isnan(AC(i)) && ~isnan(AO(i))
        ET(i) = (AC(i) - AO(i))/fs;
    else
        ET(i) = nan;
    end
    
    %IVR (MO - AC).
    if ~isnan(MO(i)) && ~isnan(AC(i))
        IVR(i) = (MO(i) - AC(i))/fs;
    else
        IVR(i) = nan;
    end
    
    % DC (T - AC) - In healthy cases, should be negative! If positive - there is diastolic contraction!
    if ecg_t(i) && ~isnan(AC(i))
        DC(i) = (ecg_t(i) - AC(i))/fs;
    else
        DC(i) = nan;
    end
    
end

IVC(1) = []; % Deleting the non-calculated first cycle (which was arbitrarily initialized to 0).
PEP(1) = []; 
ET(1) = []; 
IVR(1) = []; 
DC(1) = []; 
end

== matlab function FullCardioLablModel/SCG Analysis/Enabled SCG Analysis Subsystem/Systolic Interval Identification/Average Calculator1/slk_average_calculator ==
  data: average_type input size=[1]; series input; average output size=[1]
function average = slk_average_calculator(average_type, series)
% Simple function to return the user-defined average of an input series.

average = 0; % Pre-initialization

if average_type == 1
    average = mean(series(~isnan(series)));
elseif average_type == 2
    average = median(series(~isnan(series)));
elseif average_type == 3
    average = mode(series(~isnan(series)));
end

end

== matlab function FullCardioLablModel/SCG Analysis/Enabled SCG Analysis Subsystem/Systolic Interval Identification/Average Calculator2/slk_average_calculator ==
  data: average_type input size=[1]; series input; average output size=[1]
function average = slk_average_calculator(average_type, series)
% Simple function to return the user-defined average of an input series.

average = 0; % Pre-initialization

if average_type == 1
    average = mean(series(~isnan(series)));
elseif average_type == 2
    average = median(series(~isnan(series)));
elseif average_type == 3
    average = mode(series(~isnan(series)));
end

end

== matlab function FullCardioLablModel/ECG Analysis/Enabled ECG Analysis Subsystem/Assign To Workspace: idxs PQRST/Enabled To Workspace idxs PQRST/Slk Wrapped Assigned to Workspace ==
  data: idxs_pqrst input size=[4*ceil(param_sim_time) 5]
function slk_wrapped_assign_to_workspace(idxs_pqrst)
% Wrapped simulink function to assign an input 'assigned_var' to the base workspace.

coder.extrinsic('assign_idxs_pqrst_to_workspace');

if idxs_pqrst(:,3) % Only go into the function if a valid ECG R pos sequence is passed to it.
    assign_idxs_pqrst_to_workspace(idxs_pqrst);
end

end

== matlab function FullCardioLablModel/SCG Analysis/Enabled SCG Analysis Subsystem/Systolic Interval Identification/Average Calculator3/slk_average_calculator ==
  data: average_type input size=[1]; series input; average output size=[1]
function average = slk_average_calculator(average_type, series)
% Simple function to return the user-defined average of an input series.

average = 0; % Pre-initialization

if average_type == 1
    average = mean(series(~isnan(series)));
elseif average_type == 2
    average = median(series(~isnan(series)));
elseif average_type == 3
    average = mode(series(~isnan(series)));
end

end

== matlab function FullCardioLablModel/SCG Analysis/Enabled SCG Analysis Subsystem/Systolic Interval Identification/Average Calculator4/slk_average_calculator ==
  data: average_type input size=[1]; series input; average output size=[1]
function average = slk_average_calculator(average_type, series)
% Simple function to return the user-defined average of an input series.

average = 0; % Pre-initialization

if average_type == 1
    average = mean(series(~isnan(series)));
elseif average_type == 2
    average = median(series(~isnan(series)));
elseif average_type == 3
    average = mode(series(~isnan(series)));
end

end

== matlab function FullCardioLablModel/SCG Analysis/Enabled SCG Analysis Subsystem/Signal Generation/3D Projections/SCG xyz Average Cycle/Average SCGxyz Cycle Calculator ==
  data: r_pos input; scgxyz input; scgxyz_avgcycle output size=[3*fs 3]
function scgxyz_avgcycle  = slk_avg_scgxyz_cycle_calculator(r_pos,scgxyz)
% Simulink function to return the average x,y, and z cycles of the SCG.

% INPUTS:
% r_pos = index positions of the R peaks of the ecg.
% scgxyz = matrix of size [length_scg 3] with the (normally pre-processed) SCG
%          x,y, and z components. The first column corresponds to SCGx, the second
%          to SCGy and the third to SCGz.

% OUTPUT:
% avg_scg_xyz = matrix of size [min_rr 3] with the average SCG cycles of
%               the x,y, and z components. The first column corresponds to SCGx, the second
%               to SCGy and the third to SCGz 


% Calculating number of cycles to be considered in averaging (considered_cycles).
rr_min = min(diff(r_pos)); % Shortest cycle length - all the cycles will but cut down to this length.

if length(scgxyz) > r_pos(end) + rr_min
    considered_cycles = length(r_pos);
else
    considered_cycles = length(r_pos) - 1;
end

scg_x_cycles = zeros(rr_min,considered_cycles);
scg_y_cycles = zeros(rr_min,considered_cycles);
scg_z_cycles = zeros(rr_min,considered_cycles);

fig_scg_average_cycles = figure;

% Isolating and plotting each cycle
for i = 1:considered_cycles
    figure(fig_scg_average_cycles);
    scg_x_cycles(:,i) = scgxyz(r_pos(i):r_pos(i) + rr_min - 1,1);
    scg_y_cycles(:,i) = scgxyz(r_pos(i):r_pos(i) + rr_min - 1,2);
    scg_z_cycles(:,i) = scgxyz(r_pos(i):r_pos(i) + rr_min - 1,3);
    
    % Plotting
    subplot(3,1,1); plot(scg_x_cycles(:,i),'b'); hold on;
    subplot(3,1,2); plot(scg_y_cycles(:,i),'b'); hold on;
    subplot(3,1,3); plot(scg_z_cycles(:,i),'b'); hold on;
end

% Calculating average cycle
avg_scg_x = mean(scg_x_cycles,2);
avg_scg_y = mean(scg_y_cycles,2);
avg_scg_z = mean(scg_z_cycles,2);

% Plotting the average cycle
subplot(3,1,1); plot(avg_scg_x,'k','LineWidth',2); title('Average SCG x'); box off;
subplot(3,1,2); plot(avg_scg_y,'k','LineWidth',2); title('Average SCG y'); ylabel('Amplitude (mg)'); box off;
subplot(3,1,3); plot(avg_scg_z,'k','LineWidth',2); title('Average SCG z'); xlabel('Time (msec)'); box off;

scgxyz_avgcycle = [avg_scg_x avg_scg_y avg_scg_z];
end

== matlab function FullCardioLablModel/SCG Analysis/Enabled SCG Analysis Subsystem/Signal Generation/3D Projections/SCG xyz Average Cycle/Min RR Calculator ==
  data: r_pos input; min_rr output size=[1]
function min_rr  = slk_min_rr_calculator(r_pos)
% Simulink function to calculate the shortest RR interval from a sequence
% of R peak inputs.

% INPUTS:
% r_pos = index positions of the R peaks of the ecg.

% OUTPUT:
% min_rr = minimum RR interval.

if r_pos % Only enter the function if a valid r_pos sequence is passed to it.
    min_rr = min(diff(r_pos)); % Shortest cycle length - all the cycles will but cut down to this length.
else
    min_rr = 0;
end
end

== matlab function FullCardioLablModel/SCG Analysis/Enabled SCG Analysis Subsystem/3D Anisotropy Characterization/Average Max Diameter//Volume Calculator/Wrapped Average Max Diameter//Volume Calculator ==
  data: fs input size=[1]; r_pos input size=[4*ceil(param_sim_time) 1]; scg_xyz input size=[param_tot_samples 3]; avg_max_diameter_over_volume output size=[1]
function avg_max_diameter_over_volume = wrapped_anisotropy_calculator_avg_max_diameter_over_volume(fs,r_pos,scg_xyz) 
avg_max_diameter_over_volume=-1; % Pre-Initialization.
coder.extrinsic('anisotropy_calculator_avg_max_diameter_over_volume');
avg_max_diameter_over_volume = anisotropy_calculator_avg_max_diameter_over_volume(fs,r_pos,scg_xyz); 
end

== matlab function FullCardioLablModel/SCG Analysis/Enabled SCG Analysis Subsystem/3D Anisotropy Characterization/Average Cycle Max Diameter//Volume Calculator/Wrapped Average Cycle Max Diameter//Volume Calculator ==
  data: avg_s1_xyz input size=[0.2*fs 3]; avg_cycle_max_diameter_over_volume output size=[1]
function avg_cycle_max_diameter_over_volume = wrapped_anisotropy_calculator_avg_cycle_max_diameter_over_vol(avg_s1_xyz) 
avg_cycle_max_diameter_over_volume = -1; % Pre-Initialization.
coder.extrinsic('anisotropy_calculator_avg_cycle_max_diameter_over_volume');
avg_cycle_max_diameter_over_volume = anisotropy_calculator_avg_cycle_max_diameter_over_volume(avg_s1_xyz); 
end
